simulink model "printer01"  (Simulink 7.8)
settings: Solver=FixedStepDiscrete  StartTime=0.0  StopTime=300  FixedStep=1/2048  RelTol=1e-3
settings Model: Creator=root  LastModifiedBy=root  SimulationMode=external  ExtModeAutoUpdateStatusClock=off
settings DataIOCC: SaveOutput=off  SignalLogging=off  DSMLogging=off  SaveTime=off
settings OptimizationCC: InitFltsAndDblsToZero=on
settings DebuggingCC: SaveWithParameterizedLinksMsg=none  SignalResolutionControl=TryResolveAllWithWarning  MultiTaskDSMMsg=warning  MultiTaskCondExecSysMsg=none  FcnCallInpInsideContextMsg=Use local settings  StrictBusMsg=None
settings SFSimCC: SFSimEcho=off  SimBuildMode=sf_nonincremental_build
settings RTWCC: SystemTargetFile=ectarget.tlc  MakeCommand="make_rtw OPTS=\"-DNETIF_ID=2\""  TemplateMakefile=ec_unix.tmf  Description=Ethercattarget Real-Time Target for PREEMPT-RT/Linux  ProcessScript=ectarget_make_rtw_hook  IncludeERTFirstTime=on  RTWCompilerOptimization=On
settings CodeAppCC: GenerateComments=off  SimulinkBlockComments=off
settings GRTTargetCC: TargetFcnLib=ansi_tfl_tmw.mat  ExtMode=on

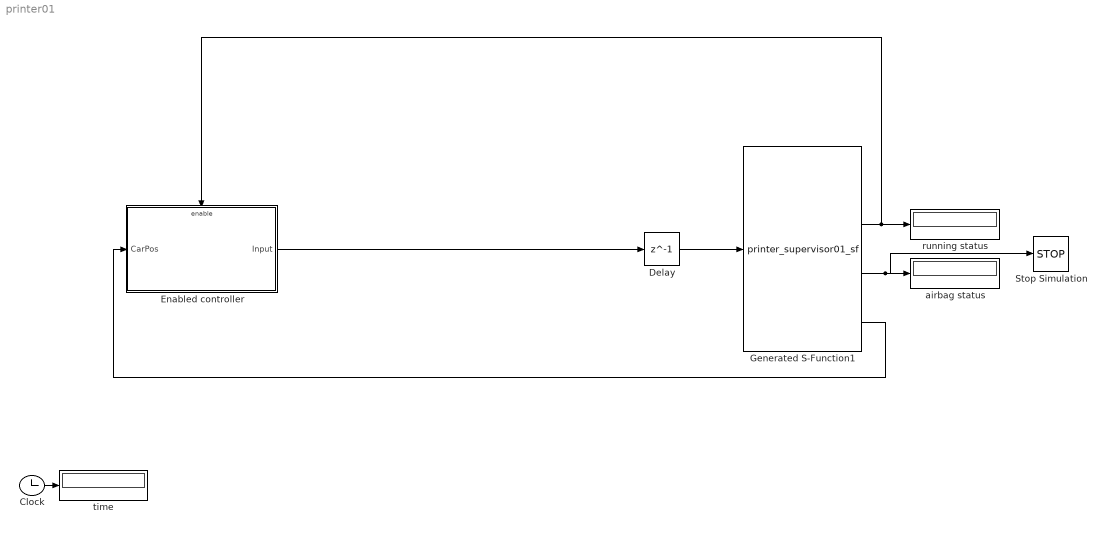
== system printer01 ==
  Clock : Clock
  Delay : Delay  DelayLength=1
  Enabled controller : Subsystem
  Generated S-Function1 : S-Function  FunctionName=printer_supervisor01_sf  SFunctionModules=""  EnableBusSupport=off  mask{rtw_sf_name=printer_supervisor01_sf, showVar=off}
      mask prompts: rtw_sf_name "Generated S-function name (model_sf):"; showVar "Show module list"
      mask help: Simulink Coder generated S-function.
      mask init:
      | displist = '';
      | if ~strcmp(get_param(gcb, 'FunctionName'), rtw_sf_name);
      |   set_param(gcb, 'FunctionName', rtw_sf_name);
      | end
      | % Check if we are generating code
      | rtw_mode = false;
      | if strcmpi(get_param(bdroot(gcb),'SimulationStatus'),'Initializing')
      | 	rtw_mode = strcmpi(get_param(bdroot(gcb),'BuildingRTWCode'),'on') && ...
      | 		~strcmpi(get_param(bdroot(gcb),'TargetStyle'),'SimulationTarget');
      | end
      | if showVar || rtw_mode
      | 	if exist('rtwsfunc') == 2 | exist('rtwsfunc') == 6
      | 		tmplist = rtwsfunc(rtw_sf_name,gcb);
      | 		tmplist = ['\nList of Modules:\n', tmplist];
      | 	elseif showVar
      | 		tmplist = '\nList of Modules:\nNot licensed\n';
      |  	end
      | end
      | if showVar
      |   displist = tmplist;
      | end
      settings: CopyFcn=|
      | if ~strcmp(get_param(gcb,'Linkstatus'),'none') && ...
      | ~strcmp(get_param(gcb,'Linkstatus'),'implicit')
      |   set_param(gcb,'LinkStatus','none');
      | end
      mask Help: eval('feval(''rtwprivate'',''rtwhelpview'',''rtw_sfcn_block'')');
      mask Display:
      | port_label('input',1,'motor [-]');
      | port_label('output',1,'time [s]');
      | port_label('output',2,'running status');
      | port_label('output',3,'airbag status');
      | port_label('output',4,'CarPos [counts]');
  Stop Simulation : Stop
  airbag status : Display
      settings: Decimation=50
  running status : Display
      settings: Decimation=50
  time : Display
      settings: Decimation=50
  wires:
  Clock/1 -> time/1
  Generated S-Function1/3 -> airbag status/1, Stop Simulation/1
  Generated S-Function1/2 -> running status/1, Enabled controller/Enable
  Generated S-Function1/4 -> Enabled controller/1(CarPos)
  Enabled controller/1(Input) -> Delay/1
  Delay/1 -> Generated S-Function1/1

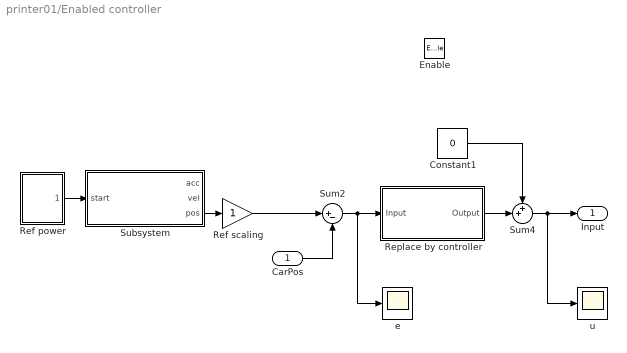
== system printer01/Enabled controller ==
  CarPos : Inport
  Enable : EnablePort
  Constant1 : Constant  Value=0
  Ref power : Subsystem  mask(On/Off Switch){stat=Off}
      mask prompts: stat "Switch"
      mask StyleString: popup(On|Off)
  "Ref scaling " : Gain  SaturateOnIntegerOverflow=on  OutDataTypeStr=Inherit: Same as input  ParamDataTypeStr=Inherit: Same as input
  Replace by controller : Subsystem
  Subsystem : Subsystem
      settings: OpenFcn=global ref_part; cb_axes 1
      mask Type: Ref3
      mask Display: disp('Ref3');
  Sum2 : Sum  Inputs=|+-
  Sum4 : Sum  Inputs=++|  SaturateOnIntegerOverflow=on  InputSameDT=on  OutDataTypeStr=Inherit: Same as first input
  e : Scope
      settings: SaveName=e  DataFormat=Array
  u : Scope
      settings: SaveName=u  DataFormat=Array
  Input : Outport
  wires:
  Sum2/1 -> e/1, Replace by controller/1(Input)
  Replace by controller/1(Output) -> Sum4/2
  Sum4/1 -> Input/1, u/1
  CarPos/1 -> Sum2/2
  Constant1/1 -> Sum4/1
  Subsystem/3(pos) -> "Ref scaling "/1
  "Ref scaling "/1 -> Sum2/1
  Ref power/1(On/Off) -> Subsystem/1(start)

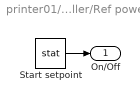
== system printer01/Enabled controller/Ref power ==
  Start setpoint : Constant  Value=stat
  On/Off : Outport
  wires:
  Start setpoint/1 -> On/Off/1

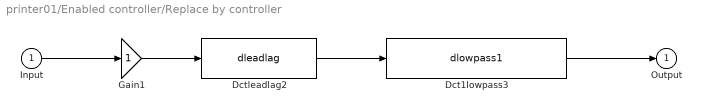
== system printer01/Enabled controller/Replace by controller ==
  Input : Inport
  Dct1lowpass3 : S-Function  FunctionName=dlowpass1  Parameters=[f_den 0.001]  EnableBusSupport=off  mask(dctools){f_den=1}
      mask prompts: f_den "Pole [Hz]"
      mask help: This block implements a discrete time 1st order lowpass filter.
      mask Display: disp('DCT 1st order lowpass')
  Dctleadlag2 : S-Function  FunctionName=dleadlag  Parameters=[f_num f_den 0.001]  EnableBusSupport=off  mask(dctools){f_num=1, f_den=1}
      mask prompts: f_num "Zero [Hz]"; f_den "Pole [Hz]"
      mask help: This block implements a discrete time leadlag filter.
      mask Display: disp('DCT leadlag')
  Gain1 : Gain  SaturateOnIntegerOverflow=on  OutDataTypeStr=Inherit: Same as input  ParamDataTypeStr=Inherit: Same as input
  Output : Outport
  wires:
  Input/1 -> Gain1/1
  Dct1lowpass3/1 -> Output/1
  Dctleadlag2/1 -> Dct1lowpass3/1
  Gain1/1 -> Dctleadlag2/1

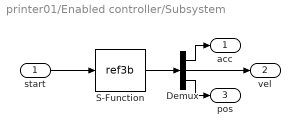
== system printer01/Enabled controller/Subsystem ==
  start : Inport
  Demux : Demux  Outputs=3
  S-Function : S-Function  FunctionName=ref3b  Parameters=ref_part  EnableBusSupport=off
      settings: OpenFcn=global ref_part; r3g_main
  acc : Outport
  vel : Outport  Port=2
  pos : Outport  Port=3
  wires:
  S-Function/1 -> Demux/1
  Demux/1 -> acc/1
  Demux/2 -> vel/1
  Demux/3 -> pos/1
  start/1 -> S-Function/1
